simulink model "Local_Partialcontrol"  (R2016a)
settings: Solver=ode8  StartTime=0.0  StopTime=800  FixedStep=1  RelTol=1e-3
settings Model: Creator=Abhiram  LastModifiedBy=Abhiram
settings GRTTargetCC: GeneratePreprocessorConditionals=Use local settings

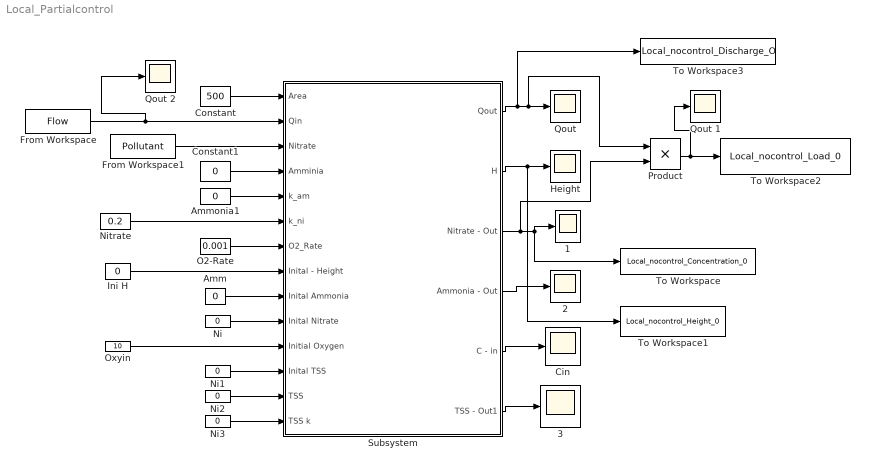
== system Local_Partialcontrol ==
  " Amm" : Constant  Value=0
  1 : Scope
  2 : Scope
  3 : Scope
  Ammonia1 : Constant  Value=0
  Cin : Scope
  Constant : Constant  Value=500
  Constant1 : Constant  Value=0
  From Workspace : FromWorkspace  VariableName=Flow  SampleTime=0
  From Workspace1 : FromWorkspace  VariableName=Pollutant  SampleTime=0
  Height : Scope
  "Ini H " : Constant  Value=0
  Ni{,1..3} (4 alike) : Constant  Value=0
  "Nitrate " : Constant  Value=0.2
  O2-Rate : Constant  Value=0.001
  "Oxyin " : Constant  Value=10
  Product : Product
  "Qout " : Scope
  Qout 1 : Scope
  Qout 2 : Scope
  Subsystem : Subsystem
  To Workspace : ToWorkspace  VariableName=Local_nocontrol_Concentration_0  SampleTime=-1
      settings: Save2DSignal=2-D array (concatenate along first dimension)
  To Workspace1 : ToWorkspace  VariableName=Local_nocontrol_Height_0  SampleTime=-1
      settings: Save2DSignal=2-D array (concatenate along first dimension)
  To Workspace2 : ToWorkspace  VariableName=Local_nocontrol_Load_0  SampleTime=-1
      settings: Save2DSignal=2-D array (concatenate along first dimension)
  To Workspace3 : ToWorkspace  VariableName=Local_nocontrol_Discharge_O  SampleTime=-1
      settings: Save2DSignal=2-D array (concatenate along first dimension)
  wires:
  "Nitrate "/1 -> Subsystem/6(k_ni)
  Constant/1 -> Subsystem/1(Area)
  From Workspace/1 -> Subsystem/2(Qin), Qout 2/1
  Ammonia1/1 -> Subsystem/5(k_am)
  Constant1/1 -> Subsystem/4(Amminia)
  From Workspace1/1 -> Subsystem/3(Nitrate)
  O2-Rate/1 -> Subsystem/7("O2_Rate ")
  Subsystem/3(Nitrate - Out) -> 1/1, To Workspace/1, Product/2
  Subsystem/4(Ammonia - Out) -> 2/1
  Subsystem/5("C - in ") -> Cin/1
  Subsystem/2(H) -> To Workspace1/1, Height/1
  "Ini H "/1 -> Subsystem/8(Inital - Height)
  " Amm"/1 -> Subsystem/9(Inital Ammonia)
  Ni/1 -> Subsystem/10(Inital Nitrate)
  "Oxyin "/1 -> Subsystem/11(Initial Oxygen)
  Subsystem/6(TSS - Out1) -> 3/1
  Ni1/1 -> Subsystem/12(Inital TSS)
  Product/1 -> Qout 1/1, To Workspace2/1
  Ni2/1 -> Subsystem/13(TSS)
  Ni3/1 -> Subsystem/14("TSS k ")
  Subsystem/1(Qout) -> To Workspace3/1, Product/1, "Qout "/1

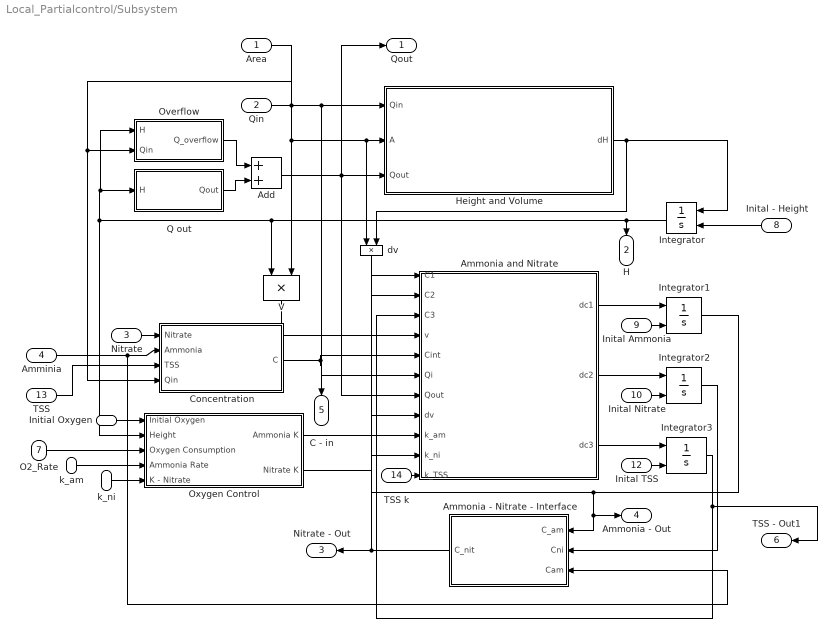
== system Local_Partialcontrol/Subsystem ==
  Area : Inport
  Qin : Inport  Port=2
  Nitrate : Inport  Port=3
  Amminia : Inport  Port=4
  k_am : Inport  Port=5
  k_ni : Inport  Port=6
  "O2_Rate " : Inport  Port=7
  Inital - Height : Inport  Port=8
  Inital Ammonia : Inport  Port=9
  Inital Nitrate : Inport  Port=10
  Initial Oxygen : Inport  Port=11
  Inital TSS : Inport  Port=12
  TSS : Inport  Port=13
  "TSS k " : Inport  Port=14
  " Ammonia - Nitrate - Interface" : MATLAB Function  TreatAsAtomicUnit=on
  " Ammonia and Nitrate " : MATLAB Function  TreatAsAtomicUnit=on
  " Concentration " : MATLAB Function  TreatAsAtomicUnit=on
  Add : Sum
  Height and Volume : MATLAB Function  TreatAsAtomicUnit=on
  Integrator : Integrator  InitialConditionSource=external  InitialCondition=10  LimitOutput=on  LowerSaturationLimit=0
  Integrator1 : Integrator  InitialConditionSource=external  LimitOutput=on  LowerSaturationLimit=0
  Integrator2 : Integrator  InitialConditionSource=external  LimitOutput=on  LowerSaturationLimit=0
  Integrator3 : Integrator  InitialConditionSource=external  LimitOutput=on  LowerSaturationLimit=0
  "Overflow " : MATLAB Function  TreatAsAtomicUnit=on
  Oxygen Control : Subsystem
  Q out : MATLAB Function  TreatAsAtomicUnit=on
  V : Product
  dv : Product
  Qout : Outport
  H : Outport  Port=2
  Nitrate - Out : Outport  Port=3
  Ammonia - Out : Outport  Port=4
  "C - in " : Outport  Port=5
  TSS - Out1 : Outport  Port=6
  wires:
  Integrator2/1 -> " Ammonia - Nitrate - Interface"/2(Cni)
  " Ammonia and Nitrate "/2(dc2) -> Integrator2/1
  " Ammonia - Nitrate - Interface"/1(C_nit) -> " Ammonia and Nitrate "/2(C2), Nitrate - Out/1
  Qin/1 -> "Overflow "/2(Qin), " Concentration "/4(Qin), " Ammonia and Nitrate "/6(Qi), Height and Volume/1(Qin)
  Height and Volume/1(dH) -> Integrator/1, dv/2
  Integrator/1 -> Oxygen Control/2(Height), Q out/1(H), "Overflow "/1(H), V/1, H/1
  Add/1 -> " Ammonia and Nitrate "/7(Qout), Qout/1, Height and Volume/3(Qout)
  Amminia/1 -> " Ammonia - Nitrate - Interface"/3(Cam), " Concentration "/2(Ammonia)
  Nitrate/1 -> " Concentration "/1(Nitrate)
  V/1 -> " Ammonia and Nitrate "/4(v)
  " Ammonia and Nitrate "/1(dc1) -> Integrator1/1
  dv/1 -> " Ammonia and Nitrate "/8(dv)
  Area/1 -> V/2, dv/1, Height and Volume/2(A)
  k_am/1 -> Oxygen Control/4("Ammonia Rate ")
  Integrator1/1 -> " Ammonia - Nitrate - Interface"/1(C_am), Ammonia - Out/1, " Ammonia and Nitrate "/1(C1)
  " Concentration "/1(C) -> " Ammonia and Nitrate "/5(Cint), "C - in "/1
  Inital Ammonia/1 -> Integrator1/2
  Inital Nitrate/1 -> Integrator2/2
  Inital - Height/1 -> Integrator/2
  Oxygen Control/2(Nitrate K) -> " Ammonia and Nitrate "/10(k_ni)
  Oxygen Control/1(Ammonia K) -> " Ammonia and Nitrate "/9(k_am)
  "O2_Rate "/1 -> Oxygen Control/3(Oxygen Consumption)
  k_ni/1 -> Oxygen Control/5(K - Nitrate)
  Initial Oxygen/1 -> Oxygen Control/1(Initial Oxygen)
  Q out/1(Qout) -> Add/2
  "Overflow "/1(Q_overflow) -> Add/1
  " Ammonia and Nitrate "/3(dc3) -> Integrator3/1
  Inital TSS/1 -> Integrator3/2
  Integrator3/1 -> TSS - Out1/1, " Ammonia and Nitrate "/3(C3)
  TSS/1 -> " Concentration "/3(TSS)
  "TSS k "/1 -> " Ammonia and Nitrate "/11(k_TSS)

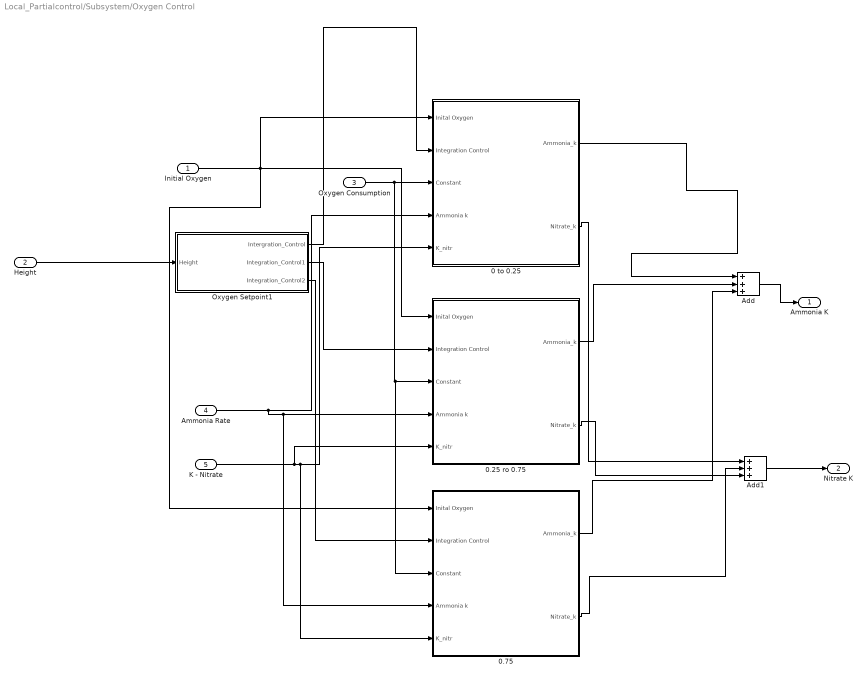
== system Local_Partialcontrol/Subsystem/Oxygen Control ==
  Initial Oxygen : Inport
  Height : Inport  Port=2
  Oxygen Consumption : Inport  Port=3
  "Ammonia Rate " : Inport  Port=4
  K - Nitrate : Inport  Port=5
  " Oxygen Setpoint1" : MATLAB Function  TreatAsAtomicUnit=on
  0 to 0.25 : Subsystem
  0.25 ro 0.75 : Subsystem
  "0.75 " : Subsystem
  Add : Sum  Inputs=3
  Add1 : Sum  Inputs=3
  Ammonia K : Outport
  Nitrate K : Outport  Port=2
  wires:
  Height/1 -> " Oxygen Setpoint1"/1(Height)
  " Oxygen Setpoint1"/2(Integration_Control1) -> 0.25 ro 0.75/2(Integration Control)
  " Oxygen Setpoint1"/1(Intergration_Control) -> 0 to 0.25/2(Integration Control)
  0 to 0.25/1(Ammonia_k) -> Add/1
  0 to 0.25/2("Nitrate_k ") -> Add1/1
  0.25 ro 0.75/1(Ammonia_k) -> Add/2
  0.25 ro 0.75/2("Nitrate_k ") -> Add1/3
  " Oxygen Setpoint1"/3(Integration_Control2) -> "0.75 "/2(Integration Control)
  Initial Oxygen/1 -> "0.75 "/1(Inital Oxygen), 0.25 ro 0.75/1(Inital Oxygen), 0 to 0.25/1(Inital Oxygen)
  Oxygen Consumption/1 -> "0.75 "/3(Constant), 0.25 ro 0.75/3(Constant), 0 to 0.25/3(Constant)
  "Ammonia Rate "/1 -> "0.75 "/4(Ammonia k), 0.25 ro 0.75/4(Ammonia k), 0 to 0.25/4(Ammonia k)
  K - Nitrate/1 -> 0.25 ro 0.75/5(K_nitr), "0.75 "/5(K_nitr), 0 to 0.25/5(K_nitr)
  "0.75 "/2("Nitrate_k ") -> Add1/2
  "0.75 "/1(Ammonia_k) -> Add/3
  Add1/1 -> Nitrate K/1
  Add/1 -> Ammonia K/1

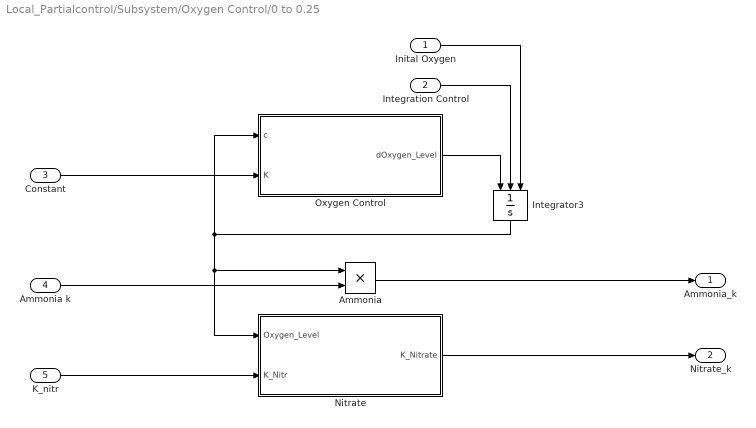
== system Local_Partialcontrol/Subsystem/Oxygen Control/0 to 0.25 ==
  Inital Oxygen : Inport
  Integration Control : Inport  Port=2
  Constant : Inport  Port=3
  Ammonia k : Inport  Port=4
  K_nitr : Inport  Port=5
  " Nitrate" : MATLAB Function  TreatAsAtomicUnit=on
  " Oxygen Control" : MATLAB Function  TreatAsAtomicUnit=on
  Ammonia : Product
  Integrator3 : Integrator  ExternalReset=level hold  InitialConditionSource=external  InitialCondition=10
  Ammonia_k : Outport
  "Nitrate_k " : Outport  Port=2
  wires:
  Inital Oxygen/1 -> Integrator3/3
  " Nitrate"/1(K_Nitrate) -> "Nitrate_k "/1
  Ammonia/1 -> Ammonia_k/1
  Ammonia k/1 -> Ammonia/2
  Constant/1 -> " Oxygen Control"/2(K)
  " Oxygen Control"/1(dOxygen_Level) -> Integrator3/1
  Integrator3/1 -> " Oxygen Control"/1(c), " Nitrate"/1(Oxygen_Level), Ammonia/1
  K_nitr/1 -> " Nitrate"/2(K_Nitr)
  Integration Control/1 -> Integrator3/2

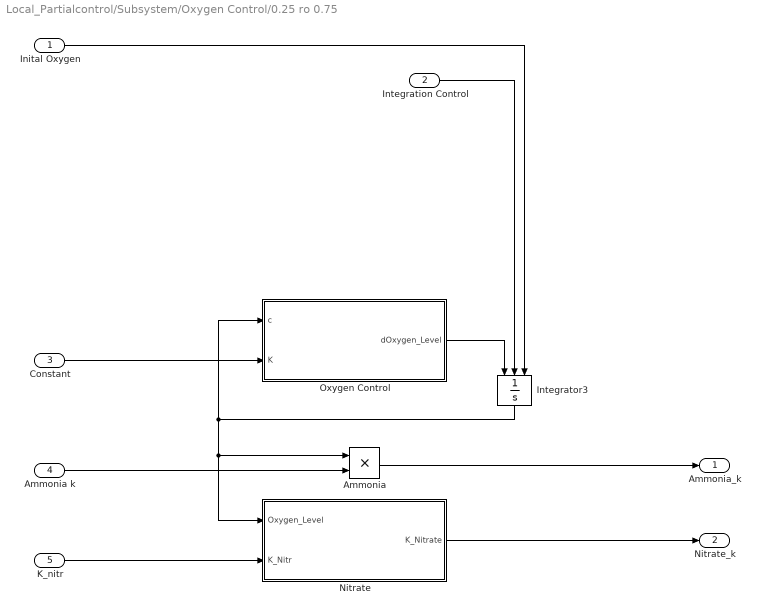
== system Local_Partialcontrol/Subsystem/Oxygen Control/0.25 ro 0.75 ==
  Inital Oxygen : Inport
  Integration Control : Inport  Port=2
  Constant : Inport  Port=3
  Ammonia k : Inport  Port=4
  K_nitr : Inport  Port=5
  " Nitrate" : MATLAB Function  TreatAsAtomicUnit=on
  " Oxygen Control" : MATLAB Function  TreatAsAtomicUnit=on
  Ammonia : Product
  Integrator3 : Integrator  ExternalReset=level hold  InitialConditionSource=external  InitialCondition=10
  Ammonia_k : Outport
  "Nitrate_k " : Outport  Port=2
  wires:
  Inital Oxygen/1 -> Integrator3/3
  " Nitrate"/1(K_Nitrate) -> "Nitrate_k "/1
  Ammonia/1 -> Ammonia_k/1
  Ammonia k/1 -> Ammonia/2
  Constant/1 -> " Oxygen Control"/2(K)
  " Oxygen Control"/1(dOxygen_Level) -> Integrator3/1
  Integrator3/1 -> " Oxygen Control"/1(c), " Nitrate"/1(Oxygen_Level), Ammonia/1
  K_nitr/1 -> " Nitrate"/2(K_Nitr)
  Integration Control/1 -> Integrator3/2

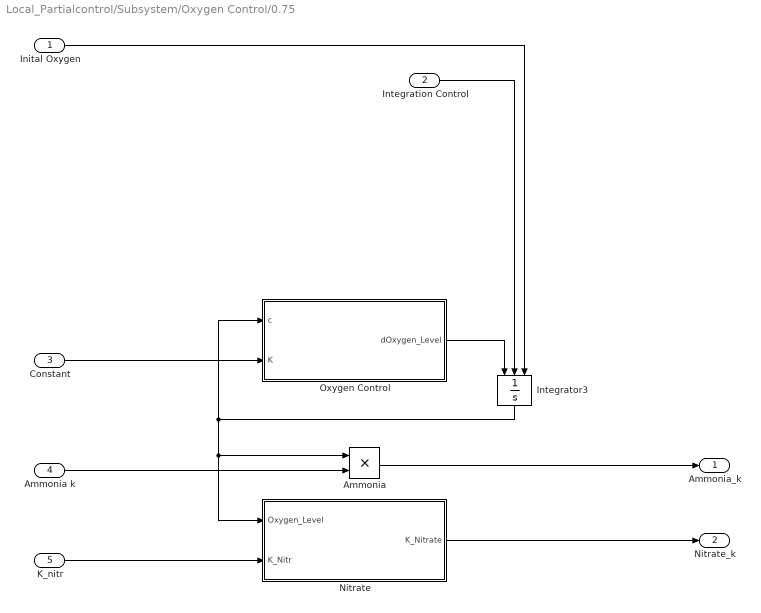
== system Local_Partialcontrol/Subsystem/Oxygen Control/0.75  ==
  Inital Oxygen : Inport
  Integration Control : Inport  Port=2
  Constant : Inport  Port=3
  Ammonia k : Inport  Port=4
  K_nitr : Inport  Port=5
  " Nitrate" : MATLAB Function  TreatAsAtomicUnit=on
  " Oxygen Control" : MATLAB Function  TreatAsAtomicUnit=on
  Ammonia : Product
  Integrator3 : Integrator  ExternalReset=level hold  InitialConditionSource=external  InitialCondition=10
  Ammonia_k : Outport
  "Nitrate_k " : Outport  Port=2
  wires:
  Inital Oxygen/1 -> Integrator3/3
  " Nitrate"/1(K_Nitrate) -> "Nitrate_k "/1
  Ammonia/1 -> Ammonia_k/1
  Ammonia k/1 -> Ammonia/2
  Constant/1 -> " Oxygen Control"/2(K)
  " Oxygen Control"/1(dOxygen_Level) -> Integrator3/1
  Integrator3/1 -> " Oxygen Control"/1(c), " Nitrate"/1(Oxygen_Level), Ammonia/1
  K_nitr/1 -> " Nitrate"/2(K_Nitr)
  Integration Control/1 -> Integrator3/2

== matlab function Local_Partialcontrol/Subsystem/Q out ==
  data: H input; Qout output
function Qout = fcn(H)

if H < 1.0
    Qout=0;
else
    Qout=2.0;
end

% Pressure head determines the discharge

== matlab function Local_Partialcontrol/Subsystem/ Ammonia - Nitrate - Interface ==
  data: C_am input; C_nit output; Cni input; Cam input
function C_nit = fcn(C_am,Cni,Cam)
C_nit=abs(C_am- Cam)+Cni;

%% Nitrate - Ammonia interface

% Nitrification converts ammonia into nitrate, which at time step is added
% to the nitrate concentration

== matlab function Local_Partialcontrol/Subsystem/ Concentration  ==
  data: Nitrate input; Ammonia input; TSS input; C output; Qin input
function C = fcn(Nitrate,Ammonia,TSS,Qin)

if Qin>0
    C=[Ammonia; Nitrate;TSS];
else
    C=[0; 0; 0];
    
end

== matlab function Local_Partialcontrol/Subsystem/Overflow  ==
  data: H input; Q_overflow output; Qin input
function Q_overflow = fcn(H,Qin)
if H>=4
    Q_overflow=Qin;
else 
    Q_overflow=0;
end

%% Function Details
% Input = Inflow, Height of the overflow wier in the pond/wetland
% Output = Discharge from overflow weir

== matlab function Local_Partialcontrol/Subsystem/Oxygen Control/ Oxygen Setpoint1 ==
  data: Height input; Intergration_Control output; Integration_Control1 output; Integration_Control2 output
function [Intergration_Control,Integration_Control1,Integration_Control2] = fcn(Height)


% Each level in pond is set with a separate integration control. O output
% ensures that integrartion happens at each time step. 1 output resets the
% integration. 

% Additional modules can be added to represent multiple division in the
% pond. Summation of cummilative value is considered to compute the total
% pollutant removal 

if Height>0 
    Intergration_Control=0; 
else 
    Intergration_Control=1;
end
    
if Height>0.25
    Integration_Control1=0;
else 
    Integration_Control1=1;
end

if Height>0.75
    Integration_Control2=0;
else 
    Integration_Control2=1;
end

== matlab function Local_Partialcontrol/Subsystem/Oxygen Control/0 to 0.25/ Nitrate ==
  data: Oxygen_Level input; K_Nitrate output; K_Nitr input
function K_Nitrate = fcn(Oxygen_Level,K_Nitr)

if Oxygen_Level< 1.0 % Set point of anoxic conditions 
    K_Nitrate = K_Nitr;
else
    K_Nitrate = 0;
end

== matlab function Local_Partialcontrol/Subsystem/Oxygen Control/0 to 0.25/ Oxygen Control ==
  data: c input; dOxygen_Level output; K input
function dOxygen_Level = fcn(c,K)

dOxygen_Level = -c * K; % First order decay of oxygen level 
end

== matlab function Local_Partialcontrol/Subsystem/Oxygen Control/0.25 ro 0.75/ Nitrate ==
  data: Oxygen_Level input; K_Nitrate output; K_Nitr input
function K_Nitrate = fcn(Oxygen_Level,K_Nitr)

if Oxygen_Level< 1.0
    K_Nitrate = K_Nitr;
else
    K_Nitrate = 0;
end

== matlab function Local_Partialcontrol/Subsystem/Oxygen Control/0.25 ro 0.75/ Oxygen Control ==
  data: c input; dOxygen_Level output; K input
function dOxygen_Level = fcn(c,K)

dOxygen_Level = -c * K;

== matlab function Local_Partialcontrol/Subsystem/Oxygen Control/0.75 / Nitrate ==
  data: Oxygen_Level input; K_Nitrate output; K_Nitr input
function K_Nitrate = fcn(Oxygen_Level,K_Nitr)

if Oxygen_Level< 1.0
    K_Nitrate = K_Nitr;
else
    K_Nitrate = 0;
end

== matlab function Local_Partialcontrol/Subsystem/ Ammonia and Nitrate  ==
  data: C1 input; C2 input; C3 input; v input; dc1 output; Cint input; Qi input; Qout input; dv input; k_am input; dc2 output; k_ni input; k_TSS input; dc3 output
function [dc1,dc2,dc3] = Nitrogen_Cycle(C1,C2,C3,v,Cint,Qi,Qout,dv,k_am,k_ni,k_TSS)

A=[Qi   0  0;
    0   Qi 0;
    0   0  Qi];

B=[Qout + dv + k_am    0               0;
    0              Qout + dv + k_ni    0;
    0                  0               Qout + dv + k_TSS ];

C=[C1;
   C2;
   C3];

if v==0 %% Ensuring 0 concentration for 0 volume 
    dc1=0;
    dc2=0;
    dc3=0;
else 
    dc=(A*Cint - B*C)*(1/v); %% CSTR equation 
    dc1=dc(1);
    dc2=dc(2);
    dc3=dc(3);

end

%% Function description 
% Input : CSTR equation data 
% Output : Change in concentration for integration

== matlab function Local_Partialcontrol/Subsystem/Oxygen Control/0.75 / Oxygen Control ==
  data: c input; dOxygen_Level output; K input
function dOxygen_Level = fcn(c,K)

dOxygen_Level = -c * K;

== matlab function Local_Partialcontrol/Subsystem/Height and Volume ==
  data: Qin input; A input; dH output; Qout input
function dH  = Height_and_Volume(Qin,A,Qout)
    dH = (Qin-Qout)*(1/A);
end

%% Function Description 

% Input : Inflow, Outflow, Area of the pond
% Output : Change in height at time step
